simulink model "dcmtr_cl_mtrReset_included"  (R2021b)
settings: Solver=ode15s  StartTime=0.0  StopTime=inf  RelTol=1e-3
undefined symbols (not defined in the file): Ts
libraries: simulink_extras x3, slpidlib x1
settings Model: Creator=smuckati  LastModifiedBy=smuckati
settings OptimizationCC: DefaultParameterBehavior=Inlined  UseDivisionForNetSlopeComputation=on  EnhancedBackFolding=on  PassReuseOutputArgsAs=Individual arguments  ZeroExternalMemoryAtStartup=off  ZeroInternalMemoryAtStartup=off  OptimizeBlockOrder=speed  DifferentSizesBufferReuse=on  OptimizationCustomize=off  EfficientTunableParamExpr=on
settings DebuggingCC: SignalRangeChecking=error  ParameterPrecisionLossMsg=none  ParameterTunabilityLossMsg=error
settings SFSimCC: MATLABDynamicMemAlloc=off
settings RTWCC: Description=Embedded Coder  SystemTargetFile=ert.tlc  GenCodeOnly=on  TemplateMakefile=ert_default_tmf  CodeExecutionProfiling=on  CodeProfilingSaveOptions=AllData  CodeProfilingInstrumentation=detailed
settings CodeAppCC: ForceParamTrailComments=on  IgnoreCustomStorageClasses=off  OperatorAnnotations=on  SimulinkDataObjDesc=on  SFDataObjDesc=on  InsertBlockDesc=on
settings ERTTargetCC: TargetLangStandard=C99 (ISO)  GenerateSampleERTMain=on  InlinedParameterPlacement=NonHierarchical  ERTCustomFileTemplate=example_file_process.tlc

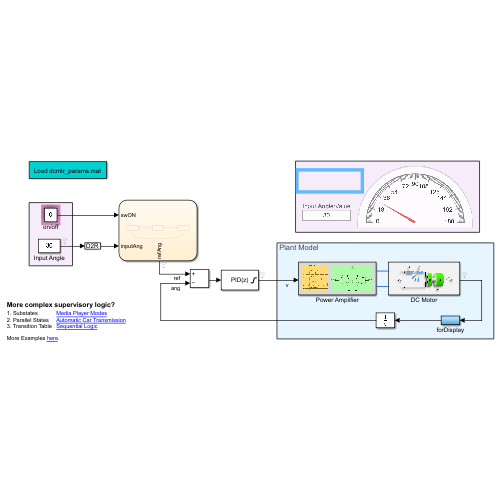
[thumbnail: Simulink's stored preview of the top-level diagram]
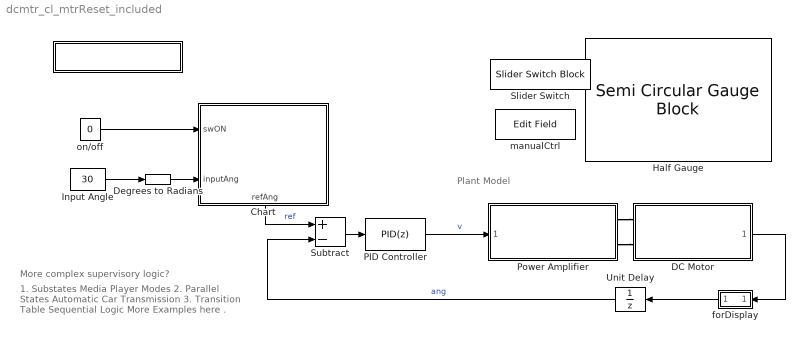
== system dcmtr_cl_mtrReset_included ==
  note: Plant Model
  note: 1. Substates Media Player Modes
      | 2. Parallel States Automatic Car Transmission
      | 3. Transition Table Sequential Logic
      |
      | More Examples here .
  note: More complex supervisory logic?
  " " : Subsystem
      settings: OpenFcn=|
      | clear
      | try
      |     load('dcmtr_params');
      |     msgbox('Variables loaded to MATLAB workspace')
      | catch
      |     error('Error loading parameters')
      | end
      mask Display: disp('Load dcmtr_params.mat')
  Chart : Stateflow chart  TreatAsAtomicUnit=on
      settings: PortSchema="{\"entries\":[{\"content\":{\"sides\":[{\"content\":{\"connectorIds\":[\"In1\",\"In2\"]},\"type\":\"ConnectorPlacement.EquallySpacedRectSide\",\"uuid\":\"8e386dd2-2ebc-4763-aebf-f59259bbb5eb\"},{\"content\":{\"connectorIds\":[],\"side\":\"RIGHT\"},\"type\":\"ConnectorPlacement.EquallySpacedRectSide\",\"uuid\":\"c3caac01-b458-4400-9120-ae3510b62e2d\"},{\"content\":{\"connectorIds\":[],\"side\":\"TOP\"},\"type\":\"ConnectorPlacement.EquallySpacedRectSide\",\"uuid\":\"fcc065d0-bf57-4436-b9d9-53a40c5b2aa1\"},{\"content\":{\"connectorIds\":[\"Out1\"],\"side\":\"BOTTOM\"},\"type\":\"ConnectorPlacement.EquallySpacedRectSide\",\"uuid\":\"e07832c5-2564-4951-b100-911dfe37d7bd\"}]},\"type\":\"ConnectorPlacement.EquallySpacedConnector\",\"uuid\":\"43767dd6-d059-4fcc-8e14-0943aede9e76\"}],\"packageUris\":[\"http://schema.mathworks.com/mf0/Connector/R2020b\"],\"version\":\"1.0\"}"
  DC Motor : Subsystem  ReferencedSubsystem=dcmtr
  Degrees to Radians : simulink_extras/Transformations/Degrees to Radians
  Half Gauge : SemiCircularGaugeBlock  LabelPosition=Hide  ScaleMax=180
  Input Angle : Constant  Value=30
  PID Controller : slpidlib/PID Controller  Controller=PID  Form=Parallel  TimeDomain=Discrete-time  UseExternalTs=off  SampleTime=Ts  IntegratorMethod=Forward Euler  FilterMethod=Forward Euler  ControllerParametersSource=internal  P=80  I=60  D=-2.214  UseFilter=on  N=7  TunerSelectOption=Transfer Function Based (PID Tuner App)  InitialConditionSource=internal  InitialConditionForIntegrator=0  InitialConditionForFilter=0  DifferentiatorICPrevScaledInput=0  ExternalReset=none  TrackingMode=off  Kt=1  LimitOutput=on  SatLimitsSource=internal  UpperSaturationLimit=5  LowerSaturationLimit=-5  LinearizeAsGain=on  AntiWindupMode=none  Kb=1  POutMin=[]  POutMax=[]  IOutMin=[]  IOutMax=[]  DOutMin=[]  DOutMax=[]  NOutMin=[]  NOutMax=[]  SumOutMin=[]  SumOutMax=[]  SaturationOutMin=[]  SaturationOutMax=[]  PParamMin=[]  PParamMax=[]  IParamMin=[]  IParamMax=[]  DParamMin=[]  DParamMax=[]  NParamMin=[]  NParamMax=[]  KbParamMin=[]  KbParamMax=[]  KtParamMin=[]  KtParamMax=[]  KbOutMin=[]  KbOutMax=[]  KtOutMin=[]  KtOutMax=[]  IntegratorOutMin=[]  IntegratorOutMax=[]  FilterOutMin=[]  FilterOutMax=[]  SumI1OutMin=[]  SumI1OutMax=[]  SumI2OutMin=[]  SumI2OutMax=[]  SumI3OutMin=[]  SumI3OutMax=[]  SumI4OutMin=[]  SumI4OutMax=[]  SumDOutMin=[]  SumDOutMax=[]  DifferentiatorOutMin=[]  DifferentiatorOutMax=[]  FilterDiffOutCoefMin=[]  FilterDiffOutCoefMax=[]  ReciprocalOutMin=[]  ReciprocalOutMax=[]  SumDenOutMin=[]  SumDenOutMax=[]  SumNumOutMin=[]  SumNumOutMax=[]  DivideOutMin=[]  DivideOutMax=[]  UdiffTsProdOutMin=[]  UdiffTsProdOutMax=[]  NTsProdOutMin=[]  NTsProdOutMax=[]  UintegralTsProdOutMin=[]  UintegralTsProdOutMax=[]  UngainTsProdOutMin=[]  UngainTsProdOutMax=[]  IntegratorContinuousStateAttributes=''  IntegratorStateMustResolveToSignalObject=off  IntegratorRTWStateStorageClass=Auto  FilterContinuousStateAttributes=''  FilterStateMustResolveToSignalObject=off  FilterRTWStateStorageClass=Auto  ParallelPVariant=InternalParameters  IdealPVariant=Disabled  IVariant=InternalParameters  DVariant=InternalParameters  IntegratorVariant=Discrete  SatVariant=Enabled  AWVariant=Passthrough  PCopyVariant=Disabled  TRVariant=Disabled  FdbkBlocksVariant=Forward  IdealPFdbkVariant=Disabled  SatFdbkVariant=Disabled  DerivativeFilterVariant=ForwardEulerFilter  NVariant=InternalParameters  NCopyVariant=Disabled  FilterICVariant=InternalICsFilter  IntegratorICVariant=InternalICs  ExternalResetVariant=Disabled  TRSumVariant=Passthrough  SumFdbkVariant=Disabled  SumVariant=Sum_PID  TsampFilterVariant=InternalTs  TsampNgainVariant=Passthrough  TsampIntegralVariant=Passthrough  ExternalSaturationOutDataTypeStr=Inherit: Same as second input
  Power Amplifier : Subsystem  ReferencedSubsystem=powerAmp
  Slider Switch : SliderSwitchBlock  LabelPosition=Hide
      settings: Values={{'zero', 'manual'}, [0 1]}
  Subtract : Sum  Inputs=+-
  Unit Delay : UnitDelay  SampleTime=Ts  HasFrameUpgradeWarning=on
  forDisplay : Subsystem
  manualCtrl : EditField  ShowInitialText=on  Alignment=Center
  on/off : Constant  Value=0  OutDataTypeStr=boolean
  wires:
  Subtract/1 -> PID Controller/1
  PID Controller/1 -> Power Amplifier/1  "v"
  Unit Delay/1 -> Subtract/2  "ang"
  Input Angle/1 -> Degrees to Radians/1
  on/off/1 -> Chart/1(swON)
  Chart/1(refAng) -> Subtract/1  "ref"
  Degrees to Radians/1 -> Chart/2(inputAng)
  DC Motor/1 -> forDisplay/1(" ")
  forDisplay/1("  ") -> Unit Delay/1
  connections:
  Power Amplifier/RConn1 -- DC Motor/LConn1
  Power Amplifier/RConn2 -- DC Motor/LConn2

== system dcmtr_cl_mtrReset_included/  ==

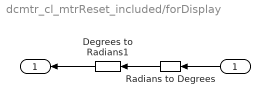
== system dcmtr_cl_mtrReset_included/forDisplay ==
  " " : Inport
  Degrees to Radians1 : simulink_extras/Transformations/Degrees to Radians
  Radians to Degrees : simulink_extras/Transformations/Radians to Degrees
  "  " : Outport
  wires:
  Radians to Degrees/1 -> Degrees to Radians1/1
  Degrees to Radians1/1 -> "  "/1
  " "/1 -> Radians to Degrees/1

== stateflow chart dcmtr_cl_mtrReset_included/Chart ==
  state mtrZERO
    refAng = 0;
  state mtrPAUSE
    refAng = 0;
  state mtrMANUAL
    refAng = inputAng;
  (default) -> mtrZERO
  mtrZERO -> mtrPAUSE : [swON == true]
  mtrPAUSE -> mtrMANUAL [order 1] : after(3,sec)
  mtrPAUSE -> mtrZERO [order 2] : [swON == false]
  mtrMANUAL -> mtrZERO : [swON == false]
  data: swON input; inputAng input; refAng output
